simulink model "casoF"  (R2018a)
settings: Solver=FixedStepAuto  StartTime=0.0  StopTime=40  RelTol=1e-3
settings Model: Creator=matth  LastModifiedBy=charlie772

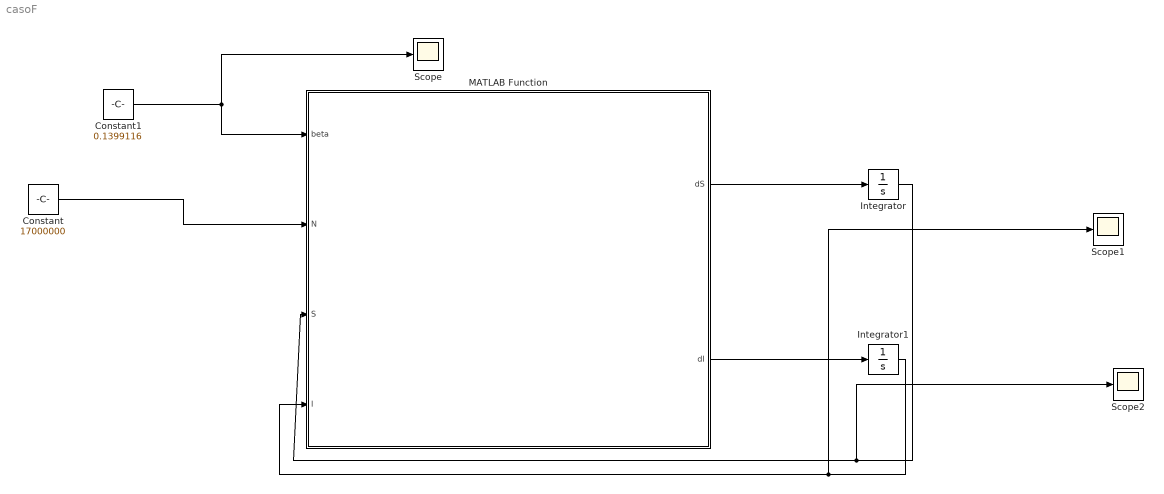
== system casoF ==
  Constant : Constant  Value=17000000
  Constant1 : Constant  Value=0.1399116
  Integrator : Integrator  InitialCondition=17000000
  Integrator1 : Integrator  InitialCondition=1
  MATLAB Function : MATLAB Function  TreatAsAtomicUnit=on
  Scope : Scope
  Scope1 : Scope
  Scope2 : Scope
  wires:
  MATLAB Function/2(dI) -> Integrator1/1
  MATLAB Function/1(dS) -> Integrator/1
  Integrator/1 -> Scope2/1, MATLAB Function/3(S)
  Integrator1/1 -> Scope1/1, MATLAB Function/4(I)
  Constant1/1 -> MATLAB Function/1(beta), Scope/1
  Constant/1 -> MATLAB Function/2(N)

== matlab function casoF/MATLAB Function ==
  data: beta input; dS output; N input; S input; I input; dI output
function [dS,dI] = SIRD(beta,N,S,I)
gamma_r = 0.0144079;
gamma_d = 0.0047093;

dS = -(beta/N)*I*S;
dI = (beta/N)*S*I - (gamma_r+gamma_d)*I; 
end
